simulink model "NN_FIT_RC_1015"  (R2023b)
settings: Solver=FixedStepAuto  StartTime=0.0  StopTime=0.1  FixedStep=1e-7  RelTol=1e-3
libraries: tiiqmathlib x9
settings Model: Creator=Jhchen  LastModifiedBy=Jhchen
settings OptimizationCC: DefaultParameterBehavior=Inlined  UseDivisionForNetSlopeComputation=on  GainParamInheritBuiltInType=on  UseFloatMulNetSlope=on  InlineInvariantSignals=on  PassReuseOutputArgsAs=Individual arguments  ZeroExternalMemoryAtStartup=off  ZeroInternalMemoryAtStartup=off  NoFixptDivByZeroProtection=on  EfficientFloat2IntCast=on  LifeSpan=1  OptimizeBlockOrder=speed  DifferentSizesBufferReuse=on  EfficientTunableParamExpr=on
settings DebuggingCC: ParameterPrecisionLossMsg=none  ParameterTunabilityLossMsg=error
settings HardwareCC: ProdBitPerChar=16  ProdBitPerInt=16  ProdBitPerPointer=32  ProdBitPerSizeT=32  ProdBitPerPtrDiffT=32  ProdLargestAtomicInteger=Integer  ProdLargestAtomicFloat=None  ProdWordSize=16  ProdLongLongMode=on  ProdHWDeviceType=Texas Instruments->C2000
settings SFSimCC: MATLABDynamicMemAlloc=off
settings RTWCC: Description=Embedded Coder  SystemTargetFile=ert.tlc  GenCodeOnly=on  TemplateMakefile=ert_default_tmf  GenerateReport=on  LaunchReport=on
settings CodeAppCC: ForceParamTrailComments=on  IgnoreCustomStorageClasses=off  OperatorAnnotations=on  SimulinkDataObjDesc=on  SFDataObjDesc=on  CustomSymbolStrGlobalVar=rt$N$M  CustomSymbolStrType=$N$M  CustomSymbolStrFcn=$N$M$F  CustomSymbolStrMacro=$N$M  InsertBlockDesc=on
settings ERTTargetCC: TargetLangStandard=C99 (ISO)  GenerateSampleERTMain=on  IncludeMdlTerminateFcn=off  CombineSignalStateStructs=on  SupportAbsoluteTime=off  SupportComplex=off  SupportNonInlinedSFcns=on  InlinedParameterPlacement=NonHierarchical  ERTCustomFileTemplate=example_file_process.tlc  ERTFilePackagingFormat=CompactWithDataFile

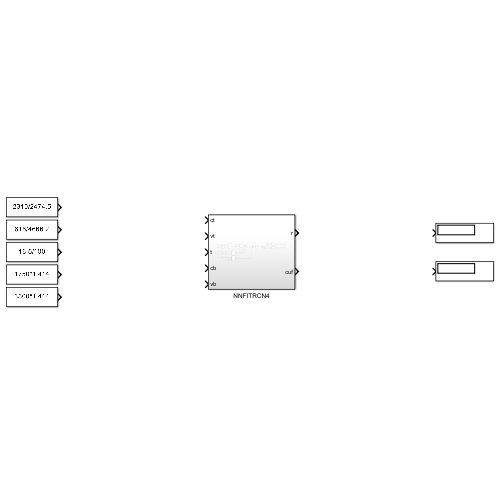
[thumbnail: Simulink's stored preview of the top-level diagram]
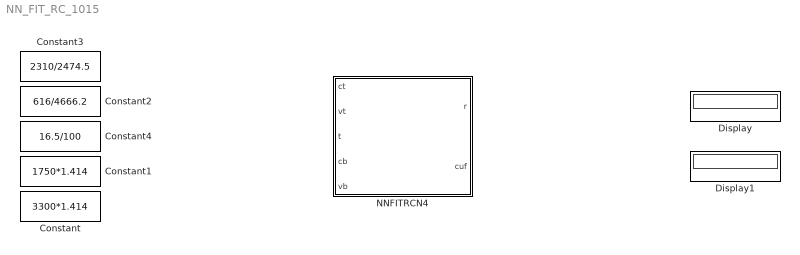
== system NN_FIT_RC_1015 ==
  Constant : Constant  Value=3300*1.414  OutDataTypeStr=single
  Constant1 : Constant  Value=1750*1.414  OutDataTypeStr=single
  Constant2 : Constant  Value=616/4666.2  OutDataTypeStr=fixdt(1,32,23)
  Constant3 : Constant  Value=2310/2474.5  OutDataTypeStr=fixdt(1,32,23)
  Constant4 : Constant  Value=16.5/100  OutDataTypeStr=fixdt(1,32,23)
  Display : Display
  Display1 : Display
  NNFITRCN4 : Subsystem

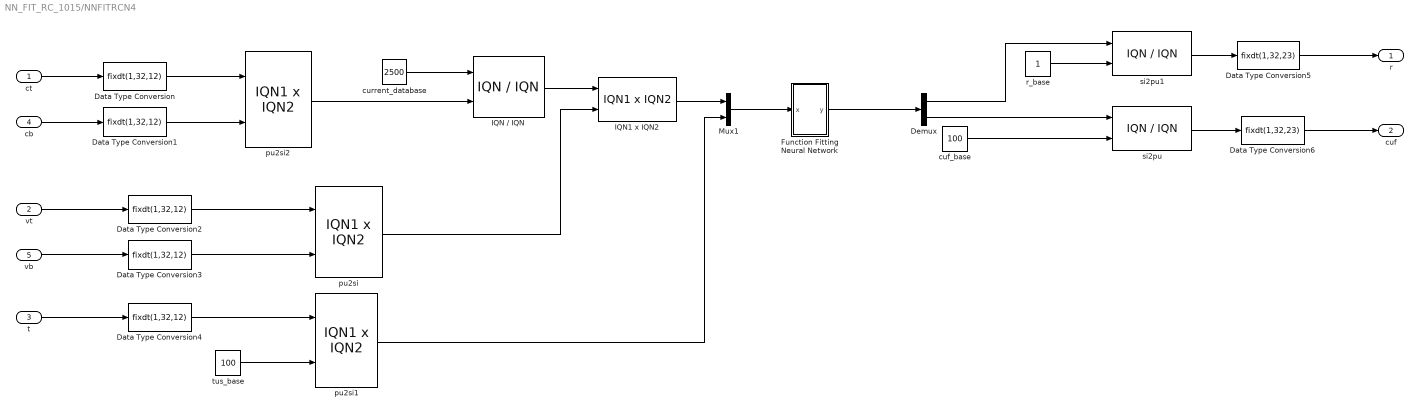
== system NN_FIT_RC_1015/NNFITRCN4 ==
  ct : Inport  OutDataTypeStr=fixdt(1,32,23)
  vt : Inport  Port=2  OutDataTypeStr=fixdt(1,32,23)
  t : Inport  Port=3  OutDataTypeStr=fixdt(1,32,23)
  cb : Inport  Port=4  OutDataTypeStr=single
  vb : Inport  Port=5  OutDataTypeStr=single
  Data Type Conversion{,1..4} (5 alike) : DataTypeConversion  OutDataTypeStr=fixdt(1,32,12)  SaturateOnIntegerOverflow=off  RndMeth=Floor
  Data Type Conversion5 : DataTypeConversion  OutDataTypeStr=fixdt(1,32,23)  SaturateOnIntegerOverflow=off  RndMeth=Floor
  Data Type Conversion6 : DataTypeConversion  OutDataTypeStr=fixdt(1,32,23)  SaturateOnIntegerOverflow=off  RndMeth=Floor
  Demux : Demux  Outputs=2
  Function Fitting Neural Network : Subsystem
  IQN / IQN : tiiqmathlib/IQN // IQN
  IQN1 x IQN2 : tiiqmathlib/IQN1 x IQN2  Q=12
  Mux1 : Mux  Inputs=2
  cuf_base : Constant  Value=100  OutDataTypeStr=fixdt(1,32,12)  LockScale=on
  current_database : Constant  Value=2500  OutDataTypeStr=fixdt(1,32,12)  LockScale=on
  pu2si : tiiqmathlib/IQN1 x IQN2  Q=12
  pu2si1 : tiiqmathlib/IQN1 x IQN2  Q=12
  pu2si2 : tiiqmathlib/IQN1 x IQN2  Q=12
  r_base : Constant  OutDataTypeStr=fixdt(1,32,12)  LockScale=on
  si2pu : tiiqmathlib/IQN // IQN
  si2pu1 : tiiqmathlib/IQN // IQN
  tus_base : Constant  Value=100  OutDataTypeStr=fixdt(1,32,12)  LockScale=on
  r : Outport  OutDataTypeStr=fixdt(1,32,23)
  cuf : Outport  Port=2  OutDataTypeStr=fixdt(1,32,23)
  wires:
  t/1 -> Data Type Conversion4/1
  Demux/1 -> si2pu1/1
  Function Fitting Neural Network/1(y) -> Demux/1
  Demux/2 -> si2pu/1
  IQN / IQN/1 -> IQN1 x IQN2/1
  Mux1/1 -> Function Fitting Neural Network/1(x)
  IQN1 x IQN2/1 -> Mux1/1
  vt/1 -> Data Type Conversion2/1
  ct/1 -> Data Type Conversion/1
  current_database/1 -> IQN / IQN/1
  cb/1 -> Data Type Conversion1/1
  vb/1 -> Data Type Conversion3/1
  pu2si/1 -> IQN1 x IQN2/2
  pu2si2/1 -> IQN / IQN/2
  Data Type Conversion/1 -> pu2si2/1
  Data Type Conversion1/1 -> pu2si2/2
  Data Type Conversion2/1 -> pu2si/1
  Data Type Conversion3/1 -> pu2si/2
  pu2si1/1 -> Mux1/2
  Data Type Conversion5/1 -> r/1
  Data Type Conversion6/1 -> cuf/1
  Data Type Conversion4/1 -> pu2si1/1
  tus_base/1 -> pu2si1/2
  cuf_base/1 -> si2pu/2
  si2pu/1 -> Data Type Conversion6/1
  r_base/1 -> si2pu1/2
  si2pu1/1 -> Data Type Conversion5/1

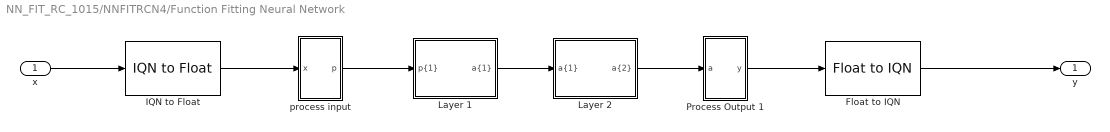
== system NN_FIT_RC_1015/NNFITRCN4/Function Fitting Neural Network ==
  x : Inport  OutDataTypeStr=fixdt(1,32,12)
  Float to IQN : tiiqmathlib/Float to IQN  Q_value=12
  IQN to Float : tiiqmathlib/IQN to Float
  Layer 1 : Subsystem
  Layer 2 : Subsystem
  Process Output 1 : Subsystem
  process input : Subsystem
  y : Outport  OutDataTypeStr=fixdt(1,32,12)  LockScale=on
  wires:
  process input/1(p) -> Layer 1/1("p{1}")
  Layer 1/1("a{1}") -> Layer 2/1("a{1}")
  Layer 2/1("a{2}") -> Process Output 1/1(a)
  x/1 -> IQN to Float/1
  Process Output 1/1(y) -> Float to IQN/1
  IQN to Float/1 -> process input/1(x)
  Float to IQN/1 -> y/1

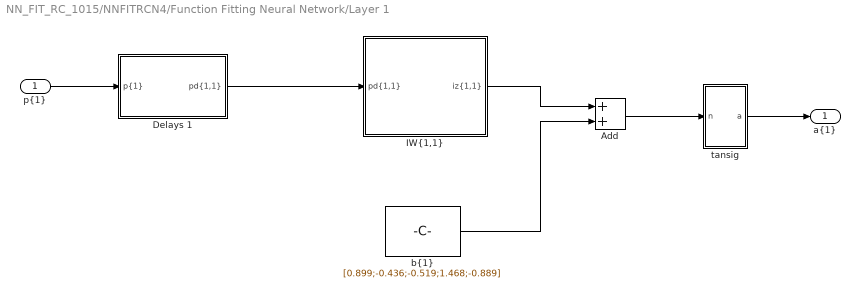
== system NN_FIT_RC_1015/NNFITRCN4/Function Fitting Neural Network/Layer 1 ==
  "p{1}" : Inport
  Add : Sum
  Delays 1 : Subsystem
  "IW{1,1}" : Subsystem
  "b{1}" : Constant  Value=[0.899;-0.436;-0.519;1.468;-0.889]  OutDataTypeStr=single
  tansig : Subsystem
  "a{1}" : Outport
  wires:
  "p{1}"/1 -> Delays 1/1("p{1}")
  tansig/1(a) -> "a{1}"/1
  Add/1 -> tansig/1(n)
  "b{1}"/1 -> Add/2
  "IW{1,1}"/1("iz{1,1}") -> Add/1
  Delays 1/1("pd{1,1}") -> "IW{1,1}"/1("pd{1,1}")

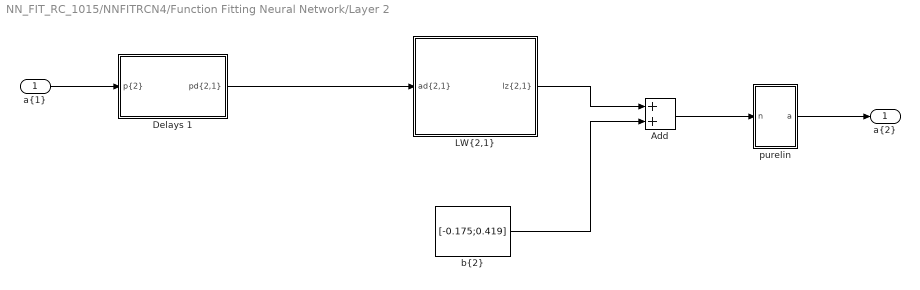
== system NN_FIT_RC_1015/NNFITRCN4/Function Fitting Neural Network/Layer 2 ==
  "a{1}" : Inport
  Add : Sum
  Delays 1 : Subsystem
  "LW{2,1}" : Subsystem
  "b{2}" : Constant  Value=[-0.175;0.419]  OutDataTypeStr=single
  purelin : Subsystem
  "a{2}" : Outport
  wires:
  Delays 1/1("pd{2,1}") -> "LW{2,1}"/1("ad{2,1}")
  "LW{2,1}"/1("lz{2,1}") -> Add/1
  "b{2}"/1 -> Add/2
  Add/1 -> purelin/1(n)
  purelin/1(a) -> "a{2}"/1
  "a{1}"/1 -> Delays 1/1("p{2}")

== system NN_FIT_RC_1015/NNFITRCN4/Function Fitting Neural Network/Process Output 1 ==
  a : Inport
  mapminmax_reverse : Subsystem
  y : Outport  VectorParamsAs1DForOutWhenUnconnected=off
  wires:
  a/1 -> mapminmax_reverse/1(y)
  mapminmax_reverse/1(x) -> y/1

== system NN_FIT_RC_1015/NNFITRCN4/Function Fitting Neural Network/process input ==
  x : Inport
  mapminmax : Subsystem
  p : Outport  VectorParamsAs1DForOutWhenUnconnected=off
  wires:
  x/1 -> mapminmax/1(x)
  mapminmax/1(y) -> p/1

== system NN_FIT_RC_1015/NNFITRCN4/Function Fitting Neural Network/Layer 1/Delays 1 ==
  "p{1}" : Inport
  Mux : Mux  Inputs=1
  "pd{1,1}" : Outport  OutDataTypeStr=single
  wires:
  "p{1}"/1 -> Mux/1
  Mux/1 -> "pd{1,1}"/1

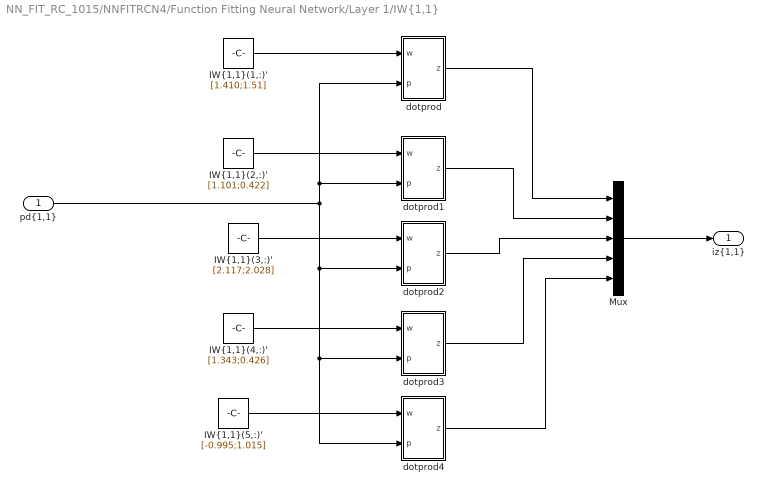
== system NN_FIT_RC_1015/NNFITRCN4/Function Fitting Neural Network/Layer 1/IW{1,1} ==
  "pd{1,1}" : Inport
  "IW{1,1}(1,:)'" : Constant  Value=[1.410;1.51]  OutDataTypeStr=single
  "IW{1,1}(2,:)'" : Constant  Value=[1.101;0.422]  OutDataTypeStr=single
  "IW{1,1}(3,:)'" : Constant  Value=[2.117;2.028]  OutDataTypeStr=single
  "IW{1,1}(4,:)'" : Constant  Value=[1.343;0.426]  OutDataTypeStr=single
  "IW{1,1}(5,:)'" : Constant  Value=[-0.995;1.015]  OutDataTypeStr=single
  Mux : Mux  Inputs=5
  dotprod : Subsystem
  dotprod1 : Subsystem
  dotprod2 : Subsystem
  dotprod3 : Subsystem
  dotprod4 : Subsystem
  "iz{1,1}" : Outport
  wires:
  Mux/1 -> "iz{1,1}"/1
  "IW{1,1}(1,:)'"/1 -> dotprod/1(w)
  "IW{1,1}(2,:)'"/1 -> dotprod1/1(w)
  "IW{1,1}(4,:)'"/1 -> dotprod3/1(w)
  dotprod1/1(z) -> Mux/2
  "IW{1,1}(5,:)'"/1 -> dotprod4/1(w)
  dotprod/1(z) -> Mux/1
  dotprod3/1(z) -> Mux/4
  dotprod2/1(z) -> Mux/3
  "pd{1,1}"/1 -> dotprod/2(p), dotprod1/2(p), dotprod2/2(p), dotprod3/2(p), dotprod4/2(p)
  dotprod4/1(z) -> Mux/5
  "IW{1,1}(3,:)'"/1 -> dotprod2/1(w)

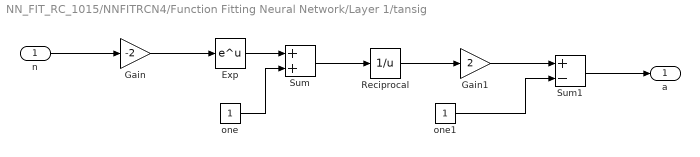
== system NN_FIT_RC_1015/NNFITRCN4/Function Fitting Neural Network/Layer 1/tansig ==
  n : Inport  OutDataTypeStr=single
  Exp : Math  SignedPower=on
  Gain : Gain  Gain=-2  SaturateOnIntegerOverflow=on  OutDataTypeStr=Inherit: Same as input  ParamDataTypeStr=Inherit: Same as input
  Gain1 : Gain  Gain=2  SaturateOnIntegerOverflow=on  OutDataTypeStr=Inherit: Same as input  ParamDataTypeStr=Inherit: Same as input
  Reciprocal : Math  Operator=reciprocal  SignedPower=on
  Sum : Sum  InputSameDT=on  SaturateOnIntegerOverflow=on  OutDataTypeStr=Inherit: Same as first input
  Sum1 : Sum  Inputs=+-  InputSameDT=on  SaturateOnIntegerOverflow=on  OutDataTypeStr=Inherit: Same as first input
  one : Constant  OutDataTypeStr=single
  one1 : Constant  OutDataTypeStr=single
  a : Outport  OutDataTypeStr=single  InitialOutput=0  VectorParamsAs1DForOutWhenUnconnected=off
  wires:
  n/1 -> Gain/1
  Sum/1 -> Reciprocal/1
  Reciprocal/1 -> Gain1/1
  Exp/1 -> Sum/1
  one/1 -> Sum/2
  Sum1/1 -> a/1
  one1/1 -> Sum1/2
  Gain/1 -> Exp/1
  Gain1/1 -> Sum1/1

== system NN_FIT_RC_1015/NNFITRCN4/Function Fitting Neural Network/Layer 2/Delays 1 ==
  "p{2}" : Inport
  Mux : Mux  Inputs=1
  "pd{2,1}" : Outport  OutDataTypeStr=single
  wires:
  Mux/1 -> "pd{2,1}"/1
  "p{2}"/1 -> Mux/1

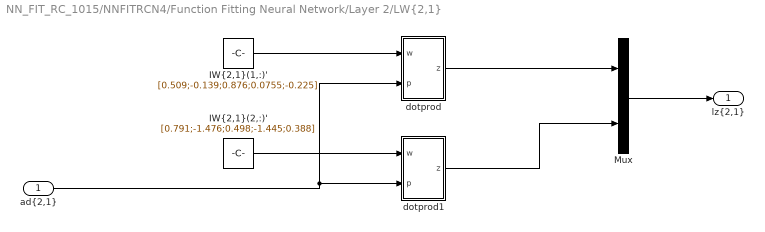
== system NN_FIT_RC_1015/NNFITRCN4/Function Fitting Neural Network/Layer 2/LW{2,1} ==
  "ad{2,1}" : Inport
  "IW{2,1}(1,:)'" : Constant  Value=[0.509;-0.139;0.876;0.0755;-0.225]  OutDataTypeStr=single
  "IW{2,1}(2,:)'" : Constant  Value=[0.791;-1.476;0.498;-1.445;0.388]  OutDataTypeStr=single
  Mux : Mux  Inputs=2
  dotprod : Subsystem
  dotprod1 : Subsystem
  "lz{2,1}" : Outport
  wires:
  "ad{2,1}"/1 -> dotprod1/2(p), dotprod/2(p)
  dotprod/1(z) -> Mux/1
  dotprod1/1(z) -> Mux/2
  "IW{2,1}(2,:)'"/1 -> dotprod1/1(w)
  "IW{2,1}(1,:)'"/1 -> dotprod/1(w)
  Mux/1 -> "lz{2,1}"/1

== system NN_FIT_RC_1015/NNFITRCN4/Function Fitting Neural Network/Layer 2/purelin ==
  n : Inport
  a : Outport  InitialOutput=0  VectorParamsAs1DForOutWhenUnconnected=off
  wires:
  n/1 -> a/1

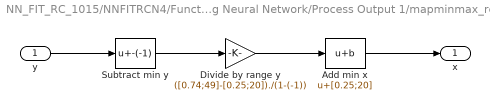
== system NN_FIT_RC_1015/NNFITRCN4/Function Fitting Neural Network/Process Output 1/mapminmax_reverse ==
  y : Inport
  Add min x : Bias  Bias=[0.25;20]  SaturateOnIntegerOverflow=off
  Divide by range y : Gain  Gain=([0.74;49]-[0.25;20])./(1-(-1))
  Subtract min y : Bias  Bias=-(-1)  SaturateOnIntegerOverflow=off
  x : Outport  VectorParamsAs1DForOutWhenUnconnected=off
  wires:
  Add min x/1 -> x/1
  Subtract min y/1 -> Divide by range y/1
  y/1 -> Subtract min y/1
  Divide by range y/1 -> Add min x/1

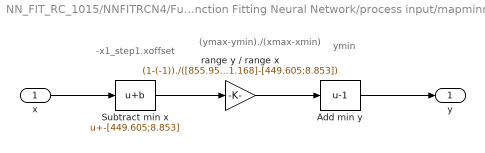
== system NN_FIT_RC_1015/NNFITRCN4/Function Fitting Neural Network/process input/mapminmax ==
  note: -x1_step1.xoffset
  note: (ymax-ymin)./(xmax-xmin)
  note: ymin
  x : Inport
  Add min y : Bias  Bias=-1  SaturateOnIntegerOverflow=off
  Subtract min x : Bias  Bias=-[449.605;8.853]
  range y / range x : Gain  Gain=(1-(-1))./([855.950;21.168]-[449.605;8.853])
  y : Outport  VectorParamsAs1DForOutWhenUnconnected=off
  wires:
  x/1 -> Subtract min x/1
  range y / range x/1 -> Add min y/1
  Add min y/1 -> y/1
  Subtract min x/1 -> range y / range x/1

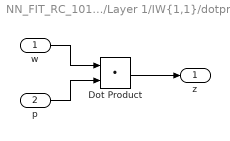
== system NN_FIT_RC_1015/NNFITRCN4/Function Fitting Neural Network/Layer 1/IW{1,1}/dotprod ==
  w : Inport
  p : Inport  Port=2
  Dot Product : DotProduct  OutDataTypeStr=Inherit: Inherit via internal rule
  z : Outport  VectorParamsAs1DForOutWhenUnconnected=off
  wires:
  Dot Product/1 -> z/1
  p/1 -> Dot Product/2
  w/1 -> Dot Product/1

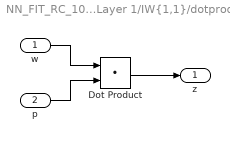
== system NN_FIT_RC_1015/NNFITRCN4/Function Fitting Neural Network/Layer 1/IW{1,1}/dotprod1 ==
  w : Inport
  p : Inport  Port=2
  Dot Product : DotProduct  OutDataTypeStr=Inherit: Inherit via internal rule
  z : Outport  VectorParamsAs1DForOutWhenUnconnected=off
  wires:
  w/1 -> Dot Product/1
  p/1 -> Dot Product/2
  Dot Product/1 -> z/1

== system NN_FIT_RC_1015/NNFITRCN4/Function Fitting Neural Network/Layer 1/IW{1,1}/dotprod2 ==
  w : Inport
  p : Inport  Port=2
  Dot Product : DotProduct  OutDataTypeStr=Inherit: Inherit via internal rule
  z : Outport  VectorParamsAs1DForOutWhenUnconnected=off
  wires:
  Dot Product/1 -> z/1
  p/1 -> Dot Product/2
  w/1 -> Dot Product/1

== system NN_FIT_RC_1015/NNFITRCN4/Function Fitting Neural Network/Layer 1/IW{1,1}/dotprod3 ==
  w : Inport
  p : Inport  Port=2
  Dot Product : DotProduct  OutDataTypeStr=Inherit: Inherit via internal rule
  z : Outport  VectorParamsAs1DForOutWhenUnconnected=off
  wires:
  w/1 -> Dot Product/1
  p/1 -> Dot Product/2
  Dot Product/1 -> z/1

== system NN_FIT_RC_1015/NNFITRCN4/Function Fitting Neural Network/Layer 1/IW{1,1}/dotprod4 ==
  w : Inport  OutDataTypeStr=single
  p : Inport  Port=2
  Dot Product : DotProduct  OutDataTypeStr=Inherit: Inherit via internal rule
  z : Outport  VectorParamsAs1DForOutWhenUnconnected=off
  wires:
  Dot Product/1 -> z/1
  p/1 -> Dot Product/2
  w/1 -> Dot Product/1

== system NN_FIT_RC_1015/NNFITRCN4/Function Fitting Neural Network/Layer 2/LW{2,1}/dotprod ==
  w : Inport
  p : Inport  Port=2
  Dot Product : DotProduct  OutDataTypeStr=Inherit: Inherit via internal rule
  z : Outport  VectorParamsAs1DForOutWhenUnconnected=off
  wires:
  w/1 -> Dot Product/1
  p/1 -> Dot Product/2
  Dot Product/1 -> z/1

== system NN_FIT_RC_1015/NNFITRCN4/Function Fitting Neural Network/Layer 2/LW{2,1}/dotprod1 ==
  w : Inport  OutDataTypeStr=single
  p : Inport  Port=2
  Dot Product : DotProduct  OutDataTypeStr=Inherit: Inherit via internal rule
  z : Outport  VectorParamsAs1DForOutWhenUnconnected=off
  wires:
  Dot Product/1 -> z/1
  p/1 -> Dot Product/2
  w/1 -> Dot Product/1
